simulink model "one_robot_hsv_nn_calibrated"  (R2024b)
settings: Solver=FixedStepDiscrete  StartTime=0.0  StopTime=20  FixedStep=0.1  MaxStep=0.1  RelTol=1e-3
libraries: realtime_pacer_lib x1
settings Model: Creator=RSL  LastModifiedBy=cwaight
settings SolverCC: AlgebraicLoopSolver=TrustRegion
settings DataIOCC: ReturnWorkspaceOutputs=off
settings DebuggingCC: UnconnectedInputMsg=warning  UnconnectedOutputMsg=warning  UnconnectedLineMsg=warning  ArithmeticOperatorsInVariantConditions=warning
settings ModelReferenceCC: EnableRefExpFcnMdlSchedulingChecks=on
settings SFSimCC: SimUseLocalCustomCode=off  CustomCodeUndefinedFunction=UseInterfaceOnly
settings RTWCC: RTWUseLocalCustomCode=off  GPUComputeCapability=3.5
settings CodeAppCC: StateflowObjectComments=on

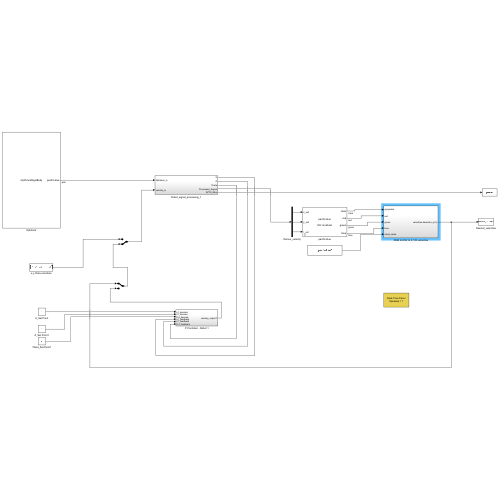
[thumbnail: Simulink's stored preview of the top-level diagram]
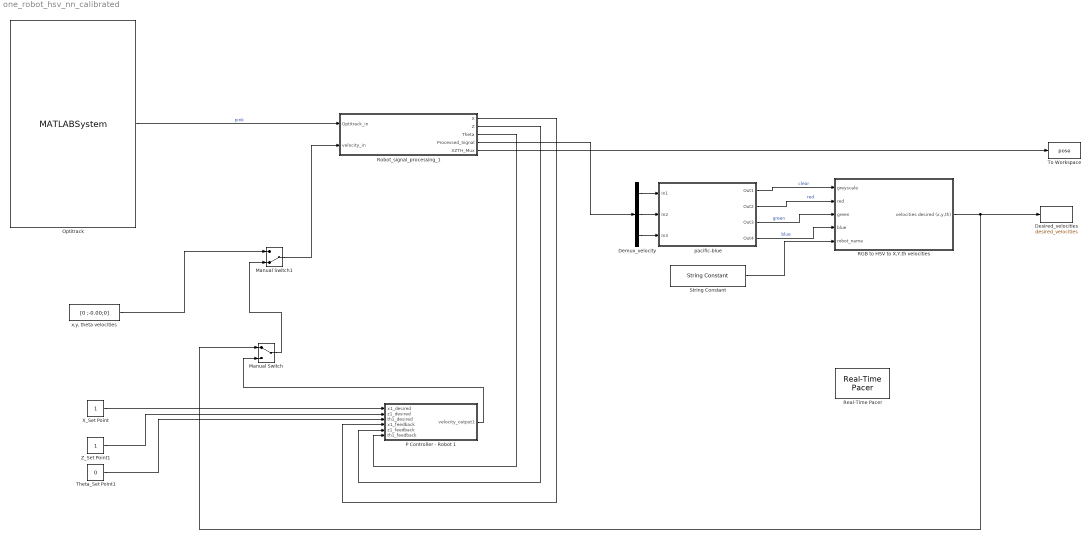
== system one_robot_hsv_nn_calibrated ==
  Demux_velocity : Demux  Outputs=3
  Desired_velocities : ToWorkspace  VariableName=desired_velocities  SampleTime=-1
  Manual Switch : ManualSwitch
  Manual Switch1 : ManualSwitch  CurrentSetting=0
  Optitrack : MATLABSystem  System=OptiTrackRigidBody  coordinateTransformationMatrix=[ 1, 0, 0; 0, 0, 1; 0, -1, 0 ]  rigidBodyNames={ 'pacific-blue'}  orientationFormat=Euler angles  debug=on  natNetHostAddress=127.0.0.1  natNetClientAddress=127.0.0.1  dllPath=C:\DecaMATLAB\NatNetSDK\lib\x64\NatNetML.dll  unicast=off
      mask Type: OptiTrackRigidBody
      mask Display:
      | disp('OptiTrackRigidBody');
      | port_label('output',1,'pacific-blue');
  P Controller - Robot 1 : Subsystem
  RGB to HSV to X,Y,th velocities : Subsystem
  Real-Time Pacer : realtime_pacer_lib/Real-Time Pacer  simTimePerRealTime=1
  Robot_signal_processing_1 : Subsystem
  String Constant : StringConstant  String="\"pacific-blue\""
  "Theta_Set Point1 " : Constant  Value=0
  To Workspace : ToWorkspace  VariableName=pose  SampleTime=-1
  X_Set Point : Constant
  Z_Set Point1 : Constant
  pacific-blue : Subsystem  mask(DecabotMask){robotName=pacific-blue, decabotHelper=localhost, robotAddress=, useDataTurbine=off, useDirectSocket=on, debug=off}
      mask prompts: robotName "Robot name:"; decabotHelper "DecabotHelper/DataTurbine server:"; robotAddress "Robot network address (optional):"; useDataTurbine "Use DataTurbine"; useDirectSocket "Use direct robot TCP connection"; debug "Log debug messages"
      mask help: This is a masked subsystem that contains a Decabot block for bidirectional communication with a decabot over a direct TCP socket connection.
      mask init:
      | robotName = 'Nobody';
      | decabotHelper = 'localhost';
      | robotAddress = '';
      | useDataTurbine = true;
      | debug = true;
      mask TypeOptions robotName: decabot/robotName
      mask Callback robotName:
      | try
      |     set_param( gcb( ), 'Name', get_param( gcb( ), 'robotName' ) );
      | end
      mask TypeOptions decabotHelper: decabot/decabotHelper
      mask TypeOptions robotAddress: decabot/robotAddress
      mask TypeOptions useDataTurbine: decabot/useDataTurbine
      mask TypeOptions useDirectSocket: decabot/useDirectSocket
      mask TypeOptions debug: decabot/debug
      mask Display:
      | disp( [get_param( gcb( ), 'robotName' ) '\n\nDH: ' get_param( gcb( ), 'decabotHelper' ) ] );
      | 
      | port_label('input',1,'x_vel');
      | port_label('input',2,'y_vel');
      | port_label('input',3,'t_vel');
      | 
      | port_label('output',1,'clear');
      | port_label('output',2,'red');
      | port_label('output',3,'green');
      | port_label('output',4,'blue');
  "x,y, theta velocities" : Constant  Value=[0 ;-0.00;0]
  wires:
  Demux_velocity/3 -> pacific-blue/3(In3)
  Demux_velocity/1 -> pacific-blue/1(In1)
  Demux_velocity/2 -> pacific-blue/2(In2)
  X_Set Point/1 -> P Controller - Robot 1/1(x1_desired)
  Z_Set Point1/1 -> P Controller - Robot 1/2(z1_desired)
  "Theta_Set Point1 "/1 -> P Controller - Robot 1/3(th1_desired)
  Robot_signal_processing_1/3(Theta) -> P Controller - Robot 1/6(th1_feedback)
  Robot_signal_processing_1/2(Z) -> P Controller - Robot 1/5(z1_feedback)
  Robot_signal_processing_1/1(X) -> P Controller - Robot 1/4(x1_feedback)
  Optitrack/1 -> Robot_signal_processing_1/1(Optitrack_in)  "pink"
  Robot_signal_processing_1/4(Processed_Signal) -> Demux_velocity/1
  pacific-blue/1(Out1) -> RGB to HSV to X,Y,th velocities/1(greyscale)  "clear"
  pacific-blue/2(Out2) -> RGB to HSV to X,Y,th velocities/2(red)  "red"
  pacific-blue/3(Out3) -> RGB to HSV to X,Y,th velocities/3(green)  "green"
  pacific-blue/4(Out4) -> RGB to HSV to X,Y,th velocities/4(blue)  "blue"
  Manual Switch1/1 -> Robot_signal_processing_1/2(velocity_in)
  P Controller - Robot 1/1(velocity_output1) -> Manual Switch/2
  Manual Switch/1 -> Manual Switch1/2
  "x,y, theta velocities"/1 -> Manual Switch1/1
  RGB to HSV to X,Y,th velocities/1(velocities desired (x,y,th)) -> Desired_velocities/1, Manual Switch/1
  Robot_signal_processing_1/5(XZTH_Mux) -> To Workspace/1
  String Constant/1 -> RGB to HSV to X,Y,th velocities/5(robot_name)

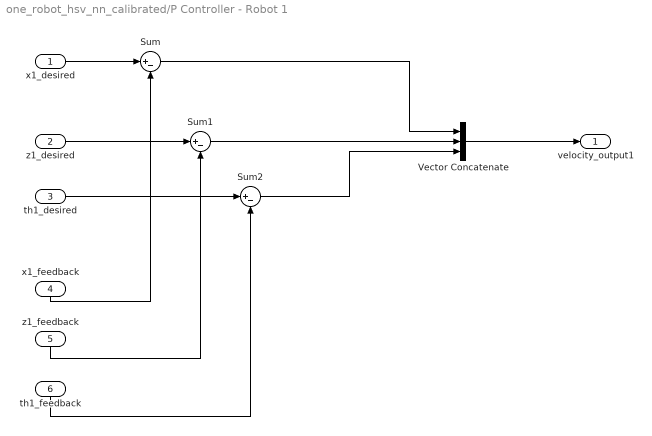
== system one_robot_hsv_nn_calibrated/P Controller - Robot 1 ==
  x1_desired : Inport
  z1_desired : Inport  Port=2
  th1_desired : Inport  Port=3
  x1_feedback : Inport  Port=4
  z1_feedback : Inport  Port=5
  th1_feedback : Inport  Port=6
  Sum : Sum  Inputs=|+-
  Sum1 : Sum  Inputs=|+-
  Sum2 : Sum  Inputs=|+-
  Vector Concatenate : Concatenate  NumInputs=3
  velocity_output1 : Outport
  wires:
  Vector Concatenate/1 -> velocity_output1/1
  x1_desired/1 -> Sum/1
  Sum/1 -> Vector Concatenate/1
  th1_feedback/1 -> Sum2/2
  x1_feedback/1 -> Sum/2
  z1_feedback/1 -> Sum1/2
  Sum2/1 -> Vector Concatenate/3
  th1_desired/1 -> Sum2/1
  Sum1/1 -> Vector Concatenate/2
  z1_desired/1 -> Sum1/1

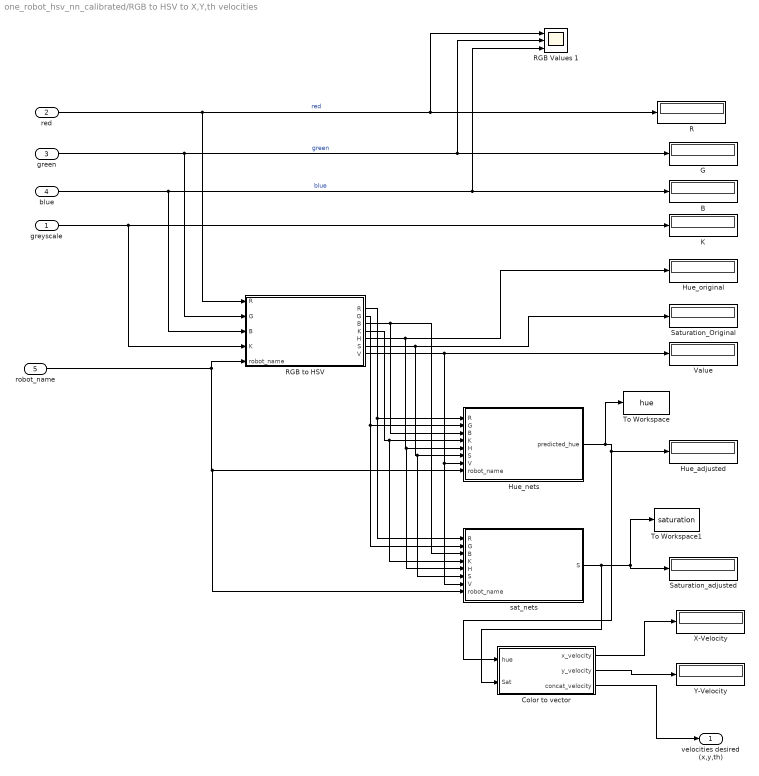
== system one_robot_hsv_nn_calibrated/RGB to HSV to X,Y,th velocities ==
  greyscale : Inport
  red : Inport  Port=2
  green : Inport  Port=3
  blue : Inport  Port=4
  robot_name : Inport  Port=5
  B : Display
  Color to vector : Subsystem
  G : Display
  Hue_adjusted : Display
  Hue_nets : MATLAB Function  TreatAsAtomicUnit=on
  Hue_original : Display
  K : Display
  R : Display
  "RGB Values 1 " : Scope  NumInputPorts=3
  RGB to HSV : MATLAB Function  TreatAsAtomicUnit=on
  Saturation_Original : Display
  Saturation_adjusted : Display
  To Workspace : ToWorkspace  VariableName=hue  SaveFormat=Timeseries  SampleTime=-1
  To Workspace1 : ToWorkspace  VariableName=saturation  SaveFormat=Timeseries  SampleTime=-1
  Value : Display
  X-Velocity : Display
  "Y-Velocity " : Display
  sat_nets : MATLAB Function  TreatAsAtomicUnit=on
  velocities desired (x,y,th) : Outport
  wires:
  red/1 -> RGB to HSV/1("R "), "RGB Values 1 "/1, R/1  "red"
  blue/1 -> "RGB Values 1 "/3, B/1, RGB to HSV/3("B ")  "blue"
  greyscale/1 -> RGB to HSV/4("K "), K/1
  green/1 -> RGB to HSV/2("G "), G/1, "RGB Values 1 "/2  "green"
  RGB to HSV/7(V) -> sat_nets/7(V), Hue_nets/7(V), Value/1
  Color to vector/3(concat_velocity) -> velocities desired (x,y,th)/1
  RGB to HSV/5(H) -> sat_nets/5(H), Hue_nets/5(H), Hue_original/1
  RGB to HSV/6(S) -> sat_nets/6("S "), Hue_nets/6(S), Saturation_Original/1
  robot_name/1 -> RGB to HSV/5(robot_name), sat_nets/8(robot_name), Hue_nets/8(robot_name)
  RGB to HSV/1(R) -> sat_nets/1(R), Hue_nets/1(R)
  RGB to HSV/2(G) -> sat_nets/2(G), Hue_nets/2(G)
  RGB to HSV/3(B) -> Hue_nets/3(B), sat_nets/3(B)
  RGB to HSV/4(K) -> sat_nets/4(K), Hue_nets/4(K)
  Hue_nets/1(predicted_hue) -> Color to vector/1(hue), Hue_adjusted/1, To Workspace/1
  sat_nets/1(S) -> Color to vector/2(Sat), To Workspace1/1, Saturation_adjusted/1
  Color to vector/1(x_velocity) -> X-Velocity/1
  Color to vector/2(y_velocity) -> "Y-Velocity "/1

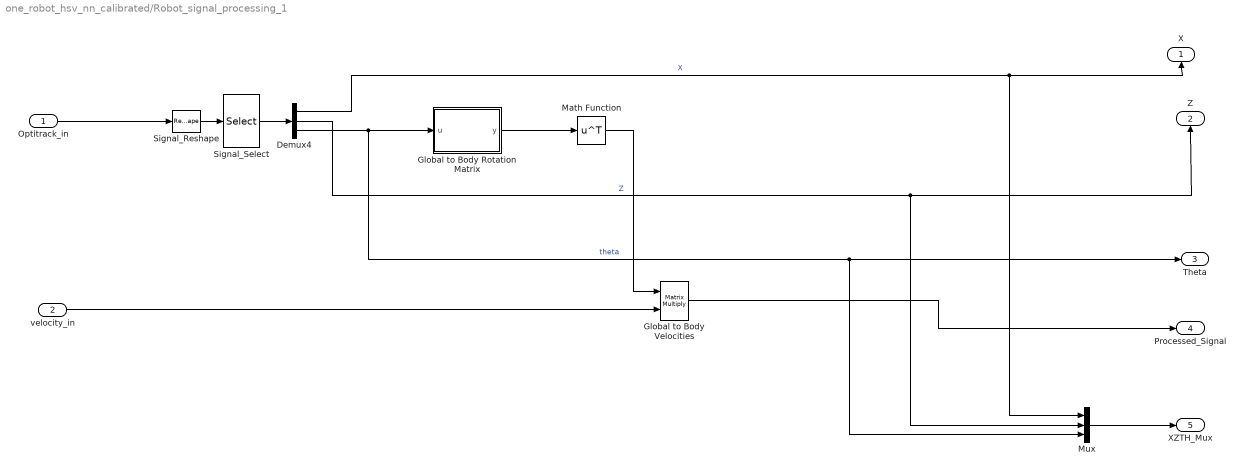
== system one_robot_hsv_nn_calibrated/Robot_signal_processing_1 ==
  Optitrack_in : Inport
  velocity_in : Inport  Port=2
  Demux4 : Demux  Outputs=3
  Global to Body Velocities : Product  Multiplication=Matrix(*)
  Global to Body Rotation Matrix : MATLAB Function  TreatAsAtomicUnit=on
  Math Function : Math  Operator=transpose  SignedPower=on
  Mux : Mux  Inputs=3
  Signal_Reshape : Reshape  OutputDimensions=6
  Signal_Select : Selector  InputPortWidth=6  IndexOptions=Index vector (dialog)  Indices=[1 2 6]  OutputSizes=1
  X : Outport
  Z : Outport  Port=2
  Theta : Outport  Port=3
  Processed_Signal : Outport  Port=4
  XZTH_Mux : Outport  Port=5
  wires:
  Demux4/1 -> Mux/1, X/1  "X"
  Demux4/3 -> Mux/3, Theta/1, Global to Body Rotation Matrix/1(u)  "theta"
  Demux4/2 -> Mux/2, Z/1  "Z"
  Global to Body Velocities/1 -> Processed_Signal/1
  Signal_Reshape/1 -> Signal_Select/1
  velocity_in/1 -> Global to Body Velocities/2
  Optitrack_in/1 -> Signal_Reshape/1
  Global to Body Rotation Matrix/1(y) -> Math Function/1
  Signal_Select/1 -> Demux4/1
  Math Function/1 -> Global to Body Velocities/1
  Mux/1 -> XZTH_Mux/1

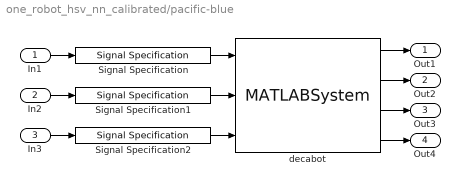
== system one_robot_hsv_nn_calibrated/pacific-blue ==
  In1 : Inport
  In2 : Inport  Port=2
  In3 : Inport  Port=3
  Signal Specification : SignalSpecification  OutDataTypeStr=double  Dimensions=1
  Signal Specification1 : SignalSpecification  OutDataTypeStr=double  Dimensions=1
  Signal Specification2 : SignalSpecification  OutDataTypeStr=double  Dimensions=1
  decabot : MATLABSystem  System=Decabot  robotName=pacific-blue  decabotHelper=localhost  useDataTurbine=off  useDirectSocket=on  debug=off
      mask Type: Decabot
      mask Display:
      | disp('pacific-blue\n\nDH: localhost');
      | port_label('input',1,'x_vel');
      | port_label('input',2,'y_vel');
      | port_label('input',3,'t_vel');
      | port_label('output',1,'clear');
      | port_label('output',2,'red');
      | port_label('output',3,'green');
      | port_label('output',4,'blue');
  Out1 : Outport
  Out2 : Outport  Port=2
  Out3 : Outport  Port=3
  Out4 : Outport  Port=4
  wires:
  Signal Specification2/1 -> decabot/3
  Signal Specification1/1 -> decabot/2
  Signal Specification/1 -> decabot/1
  In2/1 -> Signal Specification1/1
  decabot/4 -> Out4/1
  decabot/1 -> Out1/1
  decabot/3 -> Out3/1
  decabot/2 -> Out2/1
  In1/1 -> Signal Specification/1
  In3/1 -> Signal Specification2/1

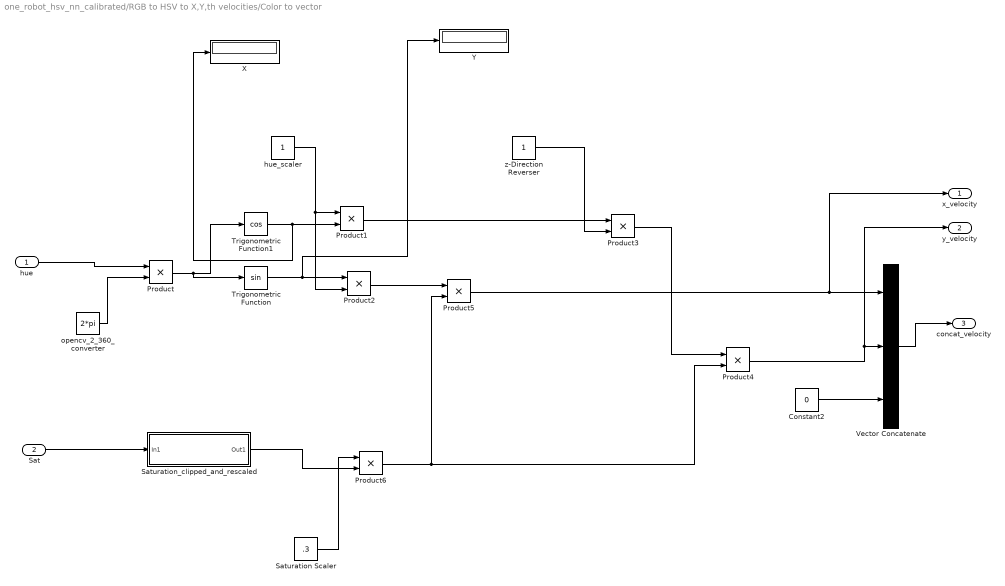
== system one_robot_hsv_nn_calibrated/RGB to HSV to X,Y,th velocities/Color to vector ==
  hue : Inport
  Sat : Inport  Port=2
  Constant2 : Constant  Value=0
  Product{,1..6} (7 alike) : Product
  Saturation Scaler : Constant  Value=.3
  Saturation_clipped_and_rescaled : Subsystem
  Trigonometric Function : Trigonometry
  Trigonometric Function1 : Trigonometry  Operator=cos
  Vector Concatenate : Concatenate  NumInputs=3
  X : Display
  Y : Display
  hue_scaler : Constant
  opencv_2_360_converter : Constant  Value=2*pi
  z-Direction Reverser : Constant
  x_velocity : Outport
  y_velocity : Outport  Port=2
  concat_velocity : Outport  Port=3
  wires:
  Trigonometric Function/1 -> Y/1, Product2/1
  opencv_2_360_converter/1 -> Product/2
  Product2/1 -> Product5/1
  Trigonometric Function1/1 -> X/1, Product1/2
  Product/1 -> Trigonometric Function1/1, Trigonometric Function/1
  Product1/1 -> Product3/1
  hue/1 -> Product/1
  hue_scaler/1 -> Product2/2, Product1/1
  Vector Concatenate/1 -> concat_velocity/1
  z-Direction Reverser/1 -> Product3/2
  Product3/1 -> Product4/1
  Product5/1 -> x_velocity/1, Vector Concatenate/1
  Constant2/1 -> Vector Concatenate/3
  Saturation Scaler/1 -> Product6/1
  Product6/1 -> Product4/2, Product5/2
  Product4/1 -> y_velocity/1, Vector Concatenate/2
  Sat/1 -> Saturation_clipped_and_rescaled/1(In1)
  Saturation_clipped_and_rescaled/1(Out1) -> Product6/2

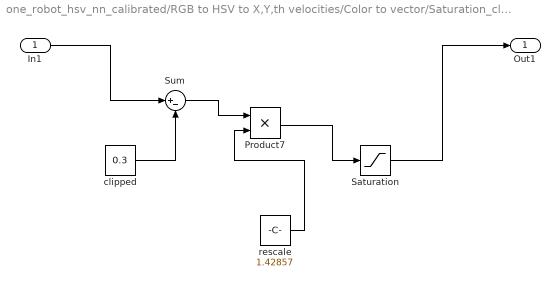
== system one_robot_hsv_nn_calibrated/RGB to HSV to X,Y,th velocities/Color to vector/Saturation_clipped_and_rescaled ==
  In1 : Inport
  Product7 : Product
  Saturation : Saturate  UpperLimit=1  LowerLimit=0.05
  Sum : Sum  Inputs=|+-
  clipped : Constant  Value=0.3
  rescale : Constant  Value=1.42857
  Out1 : Outport
  wires:
  clipped/1 -> Sum/2
  Saturation/1 -> Out1/1
  In1/1 -> Sum/1
  Product7/1 -> Saturation/1
  rescale/1 -> Product7/2
  Sum/1 -> Product7/1

== matlab function one_robot_hsv_nn_calibrated/RGB to HSV to X,Y,th velocities/RGB to HSV ==
  data: R output; G output; B output; K output; R input; H output; G input; B input; K input; S output; V output; robot_name input
function [R, G, B, K, H, S, V]= data_preprocessing(R, G, B, K, robot_name)

  if strcmp(robot_name, "celeste")  % Use strcmp for string comparison
    % Normalize RGB to [0, 1]
    R = (R - 141) / 1006;
    G = (G - 237) / 1160;
    B = (B - 241) / 1073;
    K = (K - 868) / 3032;

  elseif strcmp(robot_name, "tidal") % Use strcmp for string comparison
    % Normalize RGB to [0, 1]
    R = (R - 104) / 966;
    G = (G - 180) / 1183;
    B = (B - 174) / 1026;
    K = (K - 678) / 3021;

  elseif strcmp(robot_name, "pacific-blue") % Use strcmp for string comparison
    % Normalize RGB to [0, 1]
    R = (R - 127) / 1012;
    G = (G - 218) / 1121;
    B = (B - 219) / 971;
    K = (K - 842) / 2824;

  else  % Correct syntax for else
    % Default normalization
    R = (R - 100) / 1000;
    G = (G - 200) / 1200;
    B = (B - 200) / 1000;
    K = (K - 800) / 3000;
  end % Important: Close the if statement with "end"

  R = max(min(R, 1), 0);
  G = max(min(G, 1), 0);
  B = max(min(B, 1), 0);
  K = max(min(K, 1), 0);
  
  Cmax = max(max(R, G), B);
  Cmin = min(min(R, G), B);
  delta = Cmax - Cmin;

  H = zeros(size(R));
  S = zeros(size(R));
  V = Cmax;

  % Calculate Hue
  ind = find(delta ~= 0); 
  r_ind = find((Cmax == R) & (delta ~= 0));
  g_ind = find((Cmax == G) & (delta ~= 0));
  b_ind = find((Cmax == B) & (delta ~= 0));

  H(r_ind) = 60 * mod((G(r_ind) - B(r_ind)) ./ delta(r_ind), 6);
  H(g_ind) = 60 * (((B(g_ind) - R(g_ind)) ./ delta(g_ind)) + 2);
  H(b_ind) = 60 * (((R(b_ind) - G(b_ind)) ./ delta(b_ind)) + 4);

  H = H / 360;

  % Calculate Saturation
  S(ind) = delta(ind) ./ Cmax(ind);

end

== matlab function one_robot_hsv_nn_calibrated/RGB to HSV to X,Y,th velocities/Hue_nets ==
  data: R input; predicted_hue output; G input; B input; K input; H input; S input; V input; robot_name input
function predicted_hue = hue_nn(R, G, B, K, H, S, V, robot_name)

    % Declare persistent variables to store the networks
    persistent celeste_hue_net tidal_hue_net pacific_blue_hue_net;


    % Select the appropriate network based on robot_name
    if strcmp(robot_name, 'celeste')
        net = celeste_hue_net;
    elseif strcmp(robot_name, 'tidal')
        net = tidal_hue_net;
    elseif strcmp(robot_name, 'pacific_blue')
        net = pacific_blue_hue_net;
    else
        error('Invalid robot name');
    end

    % Create input vector
    inputs = [R, G, B, K, H, S, V]';

    % Normalize inputs to [-1, 1] using direct scaling (since we know the range is [0, 1])
    inputs = 2 * inputs - 1;

    % Get network prediction
    predicted_hue_sin_cos_normalized = net(inputs);

    % Denormalize outputs using the stored parameters (ts1_sin, ts1_cos)
    predicted_hue_sin_normalized = predicted_hue_sin_cos_normalized(1, :);
    predicted_hue_cos_normalized = predicted_hue_sin_cos_normalized(2, :);
    predicted_hue_sin = (predicted_hue_sin_normalized+1)/2;
    predicted_hue_cos = (predicted_hue_cos_normalized+1)/2;

    % Recover the hue angle using atan2
    predicted_hue = atan2(predicted_hue_sin, predicted_hue_cos) / (2 * pi);
    predicted_hue = mod(predicted_hue, 1); % Ensure it's in the range [0, 1]

end

== matlab function one_robot_hsv_nn_calibrated/RGB to HSV to X,Y,th velocities/sat_nets ==
  data: R input; S output; G input; B input; K input; H input; S input; V input; robot_name input
function S = sat_nn(R, G, B, K, H, S, V, robot_name)

    % Declare persistent variables to store the networks
    persistent celeste_sat_net tidal_sat_net pacific_blue_sat_net;


    % Select the appropriate network based on robot_name
    if strcmp(robot_name, 'celeste')
        net = celeste_sat_net;
    elseif strcmp(robot_name, 'tidal')
        net = tidal_sat_net;
    elseif strcmp(robot_name, 'pacific_blue')
        net = pacific_blue_sat_net;
    else
        error('Invalid robot name');
    end

    % Create input vector
    inputs = [R, G, B, K, H, S, V]';

    % Normalize inputs to [-1, 1] using direct scaling (since we know the range is [0, 1])
    inputs = 2 * inputs - 1;

    % Get network prediction
    predicted_sat_normalized = net(inputs);

    % Denormalize outputs using the stored parameters
    predicted_sat = (predicted_sat_normalized+1)/2;

end

== matlab function one_robot_hsv_nn_calibrated/Robot_signal_processing_1/Global to Body Rotation Matrix ==
  data: u input; y output
function y = fcn(u)

y = [cos(u) -sin(u) 0; sin(u) cos(u) 0; 0 0 1];
